simulink model "sim"  (R2024b)
settings: Solver=VariableStepAuto  StartTime=0.0  StopTime=10.0  RelTol=1e-3
values from neighbouring files (symbols this model uses):
  b1 = 2    [mFile.m]
  b2 = 2    [mFile.m]
  k1 = 3    [mFile.m]
  k2 = 4    [mFile.m]
  m1 = 2    [mFile.m]
  m2 = 1    [mFile.m]
settings Model: Creator=Ishak  LastModifiedBy=Ishak

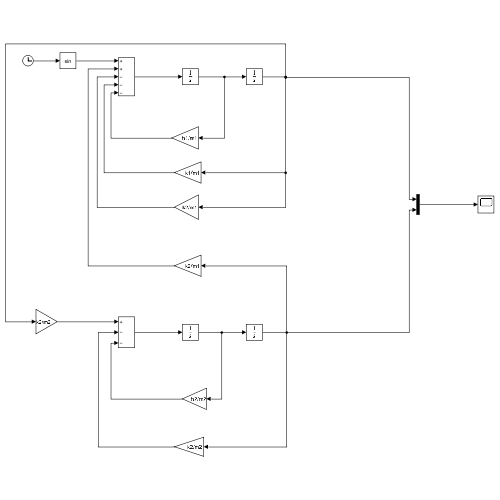
[thumbnail: Simulink's stored preview of the top-level diagram]
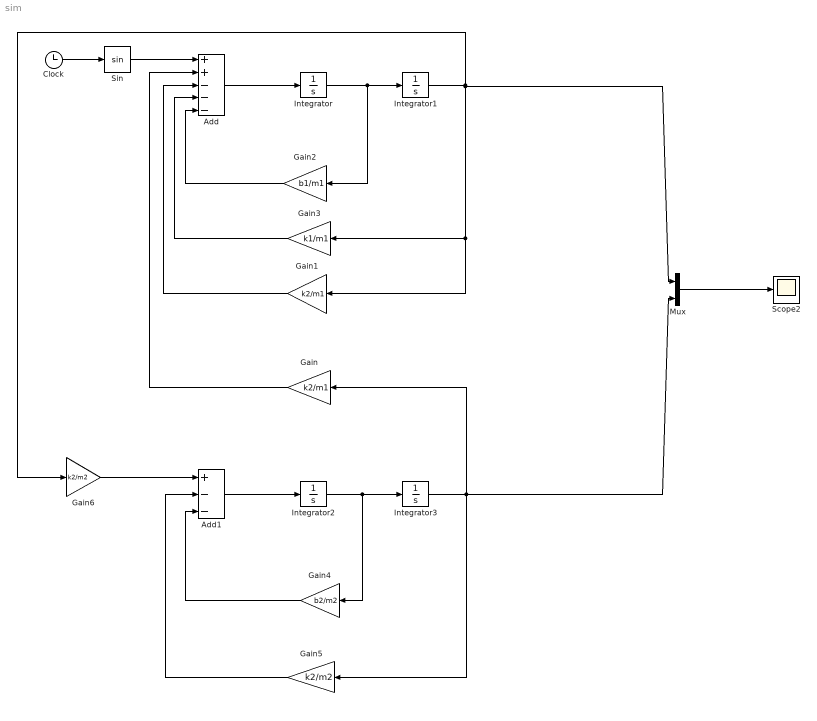
== system sim ==
  Add : Sum  Inputs=++---
  Add1 : Sum  Inputs=+--
  Clock : Clock
  Gain : Gain  Gain=k2/m1
  Gain1 : Gain  Gain=k2/m1
  Gain2 : Gain  Gain=b1/m1
  Gain3 : Gain  Gain=k1/m1
  Gain4 : Gain  Gain=b2/m2
  Gain5 : Gain  Gain=k2/m2
  Gain6 : Gain  Gain=k2/m2
  Integrator{,1..3} (4 alike) : Integrator
  Mux : Mux  Inputs=2
  Scope2 : Scope
  Sin : Trigonometry
  wires:
  Sin/1 -> Add/1
  Clock/1 -> Sin/1
  Add1/1 -> Integrator2/1
  Integrator2/1 -> Gain4/1, Integrator3/1
  Integrator3/1 -> Gain5/1, Gain/1, Mux/2
  Gain/1 -> Add/2
  Add/1 -> Integrator/1
  Integrator/1 -> Gain2/1, Integrator1/1
  Integrator1/1 -> Gain1/1, Gain3/1, Mux/1, Gain6/1
  Gain1/1 -> Add/3
  Gain2/1 -> Add/5
  Gain3/1 -> Add/4
  Mux/1 -> Scope2/1
  Gain4/1 -> Add1/3
  Gain5/1 -> Add1/2
  Gain6/1 -> Add1/1
